simulink model "simulation_discrete5"  (R2024b)
settings: Solver=FixedStepAuto  StartTime=0.0  StopTime=80  FixedStep=0.020  RelTol=1e-3
values from neighbouring files (symbols this model uses):
  output_noise_power = 0.001    [main_discrete.m]
  P0 = diag([Position_variance,Position_variance,Current_velocity_variance,Current_velocity_variance])    [main_discrete.m]
  Pb = [0.5,1]    [main_discrete.m]
  R_trajectory = 1    [main_discrete.m]
  real_inital_position = [0.5;0.3]    [main_discrete.m]
  real_vc = [0.1; 1]    [main_discrete.m]
  sim_data = struct    [main_discrete.m]
  state0_hat = [initial_x_estimate; initial_y_estimate; initial_vc_x; initial_vc_y]    [main_discrete.m]
  use_r_noise = 1    [main_discrete.m]
  use_vw_noise = 1    [main_discrete.m]
  vw_noise_power = 0.002    [main_discrete.m]
  yaw_rate = 0.2    [main_discrete.m]
libraries: simulink x3
settings Model: Creator=ricar  LastModifiedBy=ricar

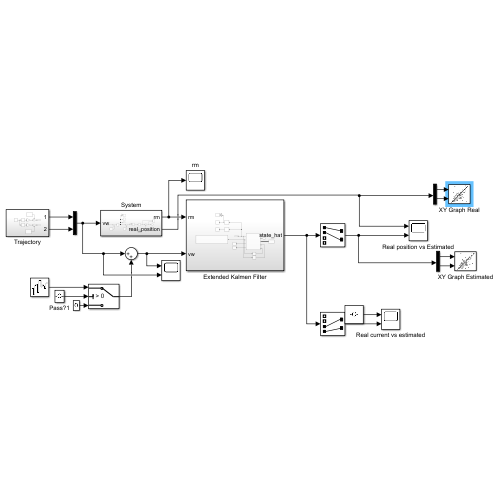
[thumbnail: Simulink's stored preview of the top-level diagram]
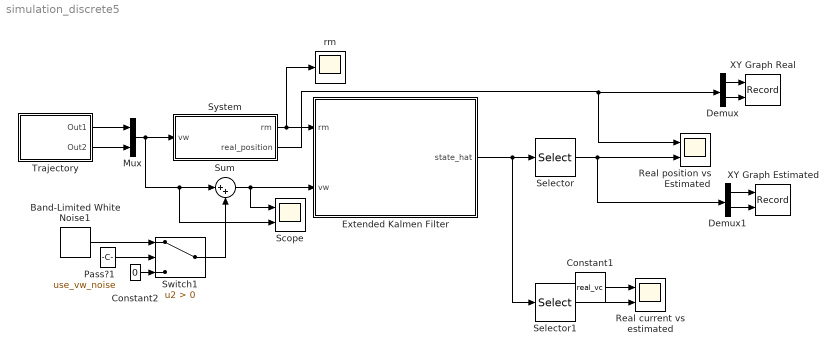
== system simulation_discrete5 ==
  Band-Limited White Noise1 : simulink/Sources/Band-Limited White Noise  Cov=[vw_noise_power,vw_noise_power]  Ts=0.1  seed=[2,3]
  Constant1 : Constant  Value=real_vc
  Constant2 : Constant  Value=0
  Demux : Demux  Outputs=2
  Demux1 : Demux  Outputs=2
  Extended Kalmen Filter : Subsystem
  Mux : Mux  Inputs=2
  Pass?1 : Constant  Value=use_vw_noise
  Real current vs estimated : Scope  NumInputPorts=2
  Real position vs Estimated : Scope  NumInputPorts=2
  Scope : Scope  NumInputPorts=2
  Selector : Selector  InputPortWidth=4  IndexOptions=Index vector (dialog)  Indices=[1 2]  OutputSizes=1
  Selector1 : Selector  InputPortWidth=4  IndexOptions=Index vector (dialog)  Indices=[3 4]  OutputSizes=1
  Sum : Sum  Inputs=|++
  Switch1 : Switch  Criteria=u2 > Threshold  SaturateOnIntegerOverflow=off  InputSameDT=off
  System : Subsystem
  Trajectory : Subsystem
  XY Graph Estimated : Record  FileSettingsInternal="{\"entries\":[{\"content\":{\"excelSettings\":{\"content\":{},\"type\":\"Streamout.ExcelSettings\"}},\"type\":\"Streamout.FileSettingStorage\",\"uuid\":\"\"}],\"packageUris\":[\"http:\\/\\/schema.mathworks.com\\/mf0\\/streamout_blocks\\/R2020a\"],\"version\":\"1.0\"}"  Layout=[1 1]  SignalsInternal="{\"entries\":[{\"content\":{\"signals\":[{\"content\":{\"blockPath\":[],\"dimensions\":[1,1],\"domain\":\"\",\"lineColor\":\"#a2142f\",\"plots\":[ 1 ],\"port\":1,\"sid\":[\"\"],\"signalID\":1,\"signalName\":\"Demux1:1\"},\"type\":\"RecordBlkView.Signal\",\"uuid\":\"\"},{\"content\":{\"blockPath\":[],\"dimensions\":[1,1],\"domain\":\"\",\"lineColor\":\"#139fff\",\"plots\":[ 1 ],\"port\":2,\"sid\":[\"\"],\"signalID\":2,\"signalName\":\"Demux1:2\"},\"type\":\"RecordBlkView.Signal\",\"uuid\":\"\"}]},\"type\":\"RecordBlkView.InputSignals\",\"uuid\":\"\"}],\"packageUris\":[\"http:\\/\\/schema.mathworks.com\\/mf0\\/streamout_blocks\\/R2020a\"],\"version\":\"1.0\"}"  VisualizationBindings="{\"xyplotplugin\":{\"info\":[{\"series\":[{\"bindingParametersList\":[{\"parameter\":\"X-Axis\",\"signalID\":1,\"signalName\":\"Demux1:1\"},{\"parameter\":\"Y-Axis\",\"signalID\":2,\"signalName\":\"Demux1:2\"}],\"seriesID\":0}],\"subplotID\":1}]}}"  CompatibilityTag=XY
  XY Graph Real : Record  FileSettingsInternal="{\"entries\":[{\"content\":{\"excelSettings\":{\"content\":{},\"type\":\"Streamout.ExcelSettings\"}},\"type\":\"Streamout.FileSettingStorage\",\"uuid\":\"\"}],\"packageUris\":[\"http:\\/\\/schema.mathworks.com\\/mf0\\/streamout_blocks\\/R2020a\"],\"version\":\"1.0\"}"  Layout=[1 1]  SignalsInternal="{\"entries\":[{\"content\":{\"signals\":[{\"content\":{\"blockPath\":[],\"dimensions\":[1],\"domain\":\"\",\"lineColor\":\"#64d413\",\"lineWidth\":2,\"plots\":[ 1 ],\"port\":1,\"sid\":[\"\"],\"signalID\":1,\"signalName\":\"Demux:1\"},\"type\":\"RecordBlkView.Signal\",\"uuid\":\"\"},{\"content\":{\"blockPath\":[],\"dimensions\":[1],\"domain\":\"\",\"lineColor\":\"#ff13a6\",\"lineWidth\":2,\"plots\":[ 1 ],\"port\":2,\"sid\":[\"\"],\"signalID\":2,\"signalName\":\"Demux:2\"},\"type\":\"RecordBlkView.Signal\",\"uuid\":\"\"}]},\"type\":\"RecordBlkView.InputSignals\",\"uuid\":\"\"}],\"packageUris\":[\"http:\\/\\/schema.mathworks.com\\/mf0\\/streamout_blocks\\/R2020a\"],\"version\":\"1.0\"}"  VisualizationBindings="{\"xyplotplugin\":{\"info\":[{\"series\":[{\"bindingParametersList\":[{\"parameter\":\"X-Axis\",\"signalID\":1,\"signalName\":\"Demux:1\"},{\"parameter\":\"Y-Axis\",\"signalID\":2,\"signalName\":\"Demux:2\"}],\"seriesID\":0}],\"subplotID\":1}]}}"  CompatibilityTag=XY
  rm : Scope
  wires:
  System/1(rm) -> rm/1, Extended Kalmen Filter/1(rm)
  Mux/1 -> Sum/1, Scope/2, System/1(vw)
  Trajectory/1(Out1) -> Mux/1
  Trajectory/2(Out2) -> Mux/2
  Extended Kalmen Filter/1(state_hat) -> Selector1/1, Selector/1
  System/2(real_position) -> Demux/1, Real position vs Estimated/1
  Selector/1 -> Demux1/1, Real position vs Estimated/2
  Selector1/1 -> Real current vs estimated/2
  Constant1/1 -> Real current vs estimated/1
  Demux1/2 -> XY Graph Estimated/2
  Demux1/1 -> XY Graph Estimated/1
  Demux/1 -> XY Graph Real/1
  Demux/2 -> XY Graph Real/2
  Switch1/1 -> Sum/2
  Pass?1/1 -> Switch1/2
  Band-Limited White Noise1/1 -> Switch1/1
  Constant2/1 -> Switch1/3
  Sum/1 -> Extended Kalmen Filter/2(vw), Scope/1

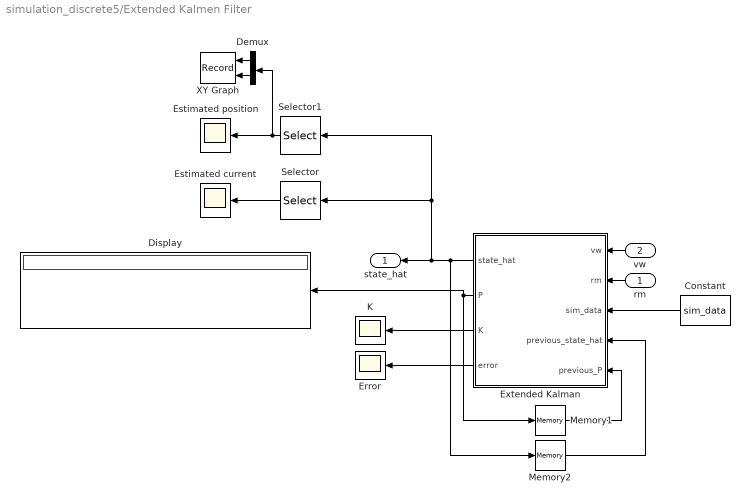
== system simulation_discrete5/Extended Kalmen Filter ==
  rm : Inport
  vw : Inport  Port=2
  Constant : Constant  Value=sim_data  OutDataTypeStr=Bus: busObject
  Demux : Demux  Outputs=2
  Display : Display
  Error : Scope
  Estimated current : Scope
  Estimated position : Scope
  Extended Kalman : MATLAB Function  TreatAsAtomicUnit=on
  K : Scope
  Memory1 : Memory  InitialCondition=P0
  Memory2 : Memory  InitialCondition=state0_hat
  Selector : Selector  InputPortWidth=4  IndexOptions=Index vector (dialog)  Indices=[3 4]  OutputSizes=1
  Selector1 : Selector  InputPortWidth=4  IndexOptions=Index vector (dialog)  Indices=[1 2]  OutputSizes=1
  XY Graph : Record  FileSettingsInternal="{\"entries\":[{\"content\":{\"excelSettings\":{\"content\":{},\"type\":\"Streamout.ExcelSettings\"}},\"type\":\"Streamout.FileSettingStorage\",\"uuid\":\"\"}],\"packageUris\":[\"http:\\/\\/schema.mathworks.com\\/mf0\\/streamout_blocks\\/R2020a\"],\"version\":\"1.0\"}"  Layout=[1 1]  SignalsInternal="{\"entries\":[{\"content\":{\"signals\":[{\"content\":{\"blockPath\":[],\"dimensions\":[1,1],\"domain\":\"\",\"lineColor\":\"#fe330a\",\"lineWidth\":2,\"plots\":[ 1 ],\"port\":1,\"sid\":[\"\"],\"signalID\":1,\"signalName\":\"Demux:1\"},\"type\":\"RecordBlkView.Signal\",\"uuid\":\"\"},{\"content\":{\"blockPath\":[],\"dimensions\":[1,1],\"domain\":\"\",\"lineColor\":\"#22b573\",\"lineWidth\":2,\"plots\":[ 1 ],\"port\":2,\"sid\":[\"\"],\"signalID\":2,\"signalName\":\"Demux:2\"},\"type\":\"RecordBlkView.Signal\",\"uuid\":\"\"}]},\"type\":\"RecordBlkView.InputSignals\",\"uuid\":\"\"}],\"packageUris\":[\"http:\\/\\/schema.mathworks.com\\/mf0\\/streamout_blocks\\/R2020a\"],\"version\":\"1.0\"}"  VisualizationBindings="{\"xyplotplugin\":{\"info\":[{\"series\":[{\"bindingParametersList\":[{\"parameter\":\"X-Axis\",\"signalID\":1,\"signalName\":\"Demux:1\"},{\"parameter\":\"Y-Axis\",\"signalID\":2,\"signalName\":\"Demux:2\"}],\"seriesID\":0},{\"bindingParametersList\":[{\"parameter\":\"X-Axis\",\"signalID\":2,\"signalName\":\"Demux:2\"}],\"seriesID\":1}],\"subplotID\":1}]}}"  CompatibilityTag=XY
  state_hat : Outport
  wires:
  vw/1 -> Extended Kalman/1(vw)
  rm/1 -> Extended Kalman/2(rm)
  Constant/1 -> Extended Kalman/3(sim_data)
  Extended Kalman/1(state_hat) -> Memory2/1, Selector1/1, Selector/1, state_hat/1
  Memory1/1 -> Extended Kalman/5(previous_P)
  Extended Kalman/2(P) -> Display/1, Memory1/1
  Memory2/1 -> Extended Kalman/4(previous_state_hat)
  Selector1/1 -> Demux/1, Estimated position/1
  Selector/1 -> Estimated current/1
  Demux/2 -> XY Graph/2
  Demux/1 -> XY Graph/1
  Extended Kalman/3(K) -> K/1
  Extended Kalman/4(error) -> Error/1

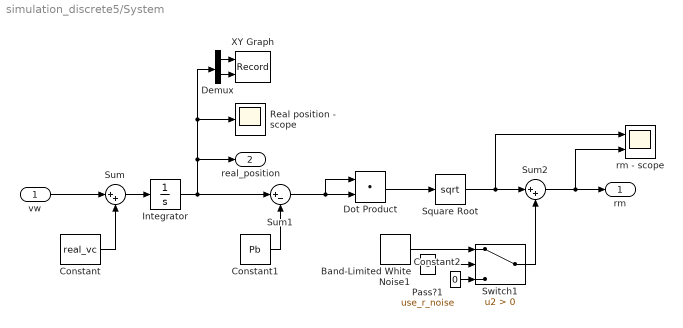
== system simulation_discrete5/System ==
  vw : Inport
  Band-Limited White Noise1 : simulink/Sources/Band-Limited White Noise  Cov=[output_noise_power]  Ts=0.1  seed=[1]
  Constant : Constant  Value=real_vc
  Constant1 : Constant  Value=Pb
  Constant2 : Constant  Value=0
  Demux : Demux  Outputs=2
  Dot Product : DotProduct  OutDataTypeStr=Inherit: Inherit via internal rule
  Integrator : Integrator  InitialCondition=real_inital_position
  Pass?1 : Constant  Value=use_r_noise
  Real position - scope : Scope
  Square Root : Sqrt
  Sum : Sum  Inputs=|++
  Sum1 : Sum  Inputs=|+-
  Sum2 : Sum  Inputs=|++
  Switch1 : Switch  Criteria=u2 > Threshold  SaturateOnIntegerOverflow=off  InputSameDT=off
  XY Graph : Record  FileSettingsInternal="{\"entries\":[{\"content\":{\"excelSettings\":{\"content\":{},\"type\":\"Streamout.ExcelSettings\"}},\"type\":\"Streamout.FileSettingStorage\",\"uuid\":\"\"}],\"packageUris\":[\"http:\\/\\/schema.mathworks.com\\/mf0\\/streamout_blocks\\/R2020a\"],\"version\":\"1.0\"}"  Layout=[1 1]  SignalsInternal="{\"entries\":[{\"content\":{\"signals\":[{\"content\":{\"blockPath\":[],\"dimensions\":[1],\"domain\":\"\",\"lineColor\":\"#0072bd\",\"lineWidth\":2,\"plots\":[ 1 ],\"port\":1,\"sid\":[\"\"],\"signalID\":1,\"signalName\":\"Demux:1\"},\"type\":\"RecordBlkView.Signal\",\"uuid\":\"\"},{\"content\":{\"blockPath\":[],\"dimensions\":[1],\"domain\":\"\",\"lineColor\":\"#d95319\",\"lineWidth\":2,\"plots\":[ 1 ],\"port\":2,\"sid\":[\"\"],\"signalID\":2,\"signalName\":\"Demux:2\"},\"type\":\"RecordBlkView.Signal\",\"uuid\":\"\"}]},\"type\":\"RecordBlkView.InputSignals\",\"uuid\":\"\"}],\"packageUris\":[\"http:\\/\\/schema.mathworks.com\\/mf0\\/streamout_blocks\\/R2020a\"],\"version\":\"1.0\"}"  VisualizationBindings="{\"xyplotplugin\":{\"info\":[{\"series\":[{\"bindingParametersList\":[{\"parameter\":\"X-Axis\",\"signalID\":1,\"signalName\":\"Demux:1\"},{\"parameter\":\"Y-Axis\",\"signalID\":2,\"signalName\":\"Demux:2\"}],\"seriesID\":0}],\"subplotID\":1}]}}"  CompatibilityTag=XY
  rm - scope : Scope  NumInputPorts=2
  rm : Outport
  real_position : Outport  Port=2
  wires:
  vw/1 -> Sum/1
  Constant/1 -> Sum/2
  Sum/1 -> Integrator/1
  Integrator/1 -> real_position/1, Real position - scope/1, Demux/1, Sum1/1
  Constant1/1 -> Sum1/2
  Square Root/1 -> Sum2/1, rm - scope/1
  Sum1/1 -> Dot Product/1, Dot Product/2
  Dot Product/1 -> Square Root/1
  Demux/1 -> XY Graph/1
  Demux/2 -> XY Graph/2
  Switch1/1 -> Sum2/2
  Constant2/1 -> Switch1/3
  Band-Limited White Noise1/1 -> Switch1/1
  Pass?1/1 -> Switch1/2
  Sum2/1 -> rm/1, rm - scope/2

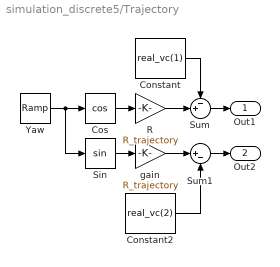
== system simulation_discrete5/Trajectory ==
  Constant : Constant  Value=real_vc(1)
  Constant2 : Constant  Value=real_vc(2)
  Cos : Trigonometry  Operator=cos
  R : Gain  Gain=R_trajectory
  Sin : Trigonometry
  Sum : Sum  Inputs=-+|
  Sum1 : Sum  Inputs=|+-
  Yaw : simulink/Sources/Ramp  slope=yaw_rate  start=0  InitialOutput=0
  gain : Gain  Gain=R_trajectory
  Out1 : Outport
  Out2 : Outport  Port=2
  wires:
  Cos/1 -> R/1
  gain/1 -> Sum1/1
  R/1 -> Sum/2
  Yaw/1 -> Cos/1, Sin/1
  Constant2/1 -> Sum1/2
  Constant/1 -> Sum/1
  Sin/1 -> gain/1
  Sum1/1 -> Out2/1
  Sum/1 -> Out1/1

== matlab function simulation_discrete5/Extended Kalmen Filter/Extended Kalman ==
  data: vw input; rm input; sim_data input; state_hat output; previous_state_hat input; previous_P input; P output; K output; error output
function [state_hat, P, K,error] = fcn(vw,rm,sim_data,previous_state_hat,previous_P)

% Initialize variable from workspace
    % Known:
    Pb = sim_data.Beacon_position;

    % System dynamics
    F = sim_data.F;
    G = sim_data.G;

    % Cant bring from sim_data due to matlab complications
    h = @(x,y) sqrt((x-Pb(1))^2 + (y-Pb(2))^2);

    J_h = @(x_hat,y_hat,v_cx,v_c) [(x_hat-Pb(1))/h(x_hat,y_hat), ...
                      (y_hat-Pb(2))/h(x_hat,y_hat), ...
                      0, ...
                      0];

    % Filter initiation
    Q = sim_data.state_noise;
    R = sim_data.measurement_noise;

%% Extended Kalmen Filter Logic

% Prediction
prediction_P = F * previous_P * F.'+ Q;
state_prediction = F*previous_state_hat + G * vw; 

x_hat = state_prediction(1);
y_hat = state_prediction(2);
v_cx_hat = state_prediction(3);
v_cy_hat = state_prediction(4);

output_prediction = h(x_hat,y_hat);

    % Calculate H matrix from current estimate
H = J_h(x_hat,y_hat,v_cx_hat,v_cy_hat);

% Update
K = prediction_P * H.' * (H * prediction_P * H.' + R)^(-1);

error = rm-output_prediction;
state_hat = state_prediction + K*error;

I = eye(4);
P = (I - K * H)* prediction_P;
